simulink model "Pendel"  (Simulink 8.1)
settings: Solver=ode45  StartTime=0.0  StopTime=10.0  RelTol=1e-3
values from neighbouring files (symbols this model uses):
  dphi0 = 0    [Aufgabe_7_Loesung.m]
  dx0 = 0    [Aufgabe_7_Loesung.m]
  g = 9.81    [Aufgabe_7_Loesung.m]    (also in Aufgabe_8_Loesung.m)
  J_d = 5.8134e-4    (= 0.00058134)    [Aufgabe_7_Loesung.m]    (also in Aufgabe_8_Loesung.m)
  K = 1    [Aufgabe_7_Loesung.m]    (also in Aufgabe_8_Loesung.m)
  l_p = 0.147    [Aufgabe_7_Loesung.m]    (also in Aufgabe_8_Loesung.m)
  l_s = 0.5    [Aufgabe_7_Loesung.m]    (also in Aufgabe_8_Loesung.m)
  m_p = 0.0804    [Aufgabe_7_Loesung.m]    (also in Aufgabe_8_Loesung.m)
  mu = 8.5e-6    (= 8.5e-06)    [Aufgabe_7_Loesung.m]    (also in Aufgabe_8_Loesung.m)
  phi0 = 0    [Aufgabe_7_Loesung.m]
  T1 = 0.043    [Aufgabe_7_Loesung.m]    (also in Aufgabe_8_Loesung.m)
  Tt = 0.03    [Aufgabe_7_Loesung.m]    (also in Aufgabe_8_Loesung.m)
  x0 = 0    [Aufgabe_7_Loesung.m]
settings Model: Creator=St  LastModifiedBy=St
settings DataIOCC: SignalLoggingSaveFormat=Dataset
settings OptimizationCC: ExpressionDepthLimit=128
settings DebuggingCC: FcnCallInpInsideContextMsg=EnableAllAsError
settings GRTTargetCC: CombineOutputUpdateFcns=on  GRTInterface=off

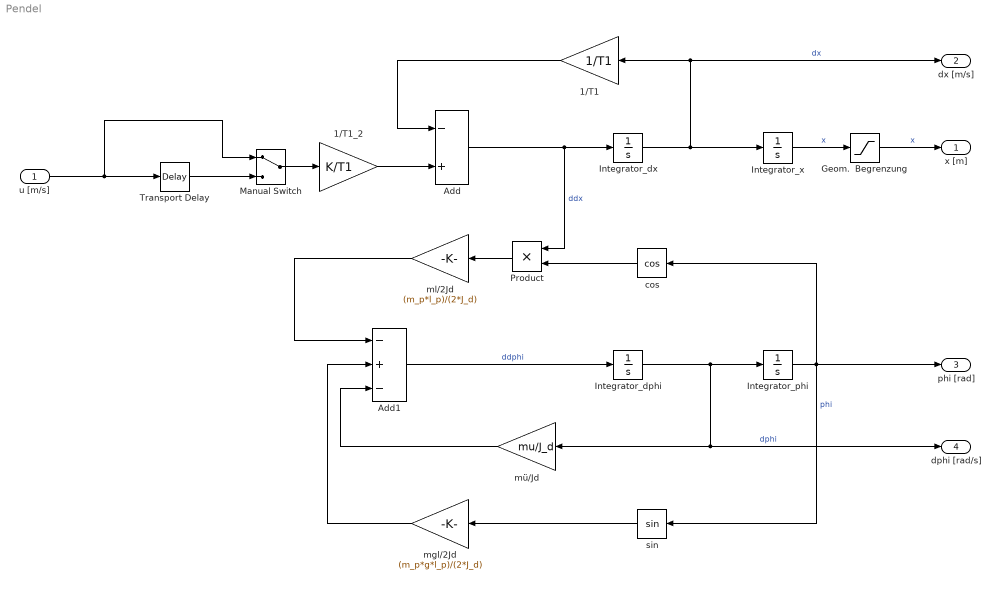
== system Pendel ==
  u [m/s] : Inport
  1/T1 : Gain  Gain=1/T1
  1/T1_2 : Gain  Gain=K/T1
  Add : Sum  Inputs=-+
  Add1 : Sum  Inputs=-+-
  Geom.  Begrenzung : Saturate  UpperLimit=l_s/2  LowerLimit=-l_s/2
  Integrator_dphi : Integrator  InitialCondition=dphi0
  Integrator_dx : Integrator  InitialCondition=dx0
  Integrator_phi : Integrator  InitialCondition=phi0
  Integrator_x : Integrator  InitialCondition=x0  UpperSaturationLimit=l_s/2  LowerSaturationLimit=-l_s/2
  Manual Switch : ManualSwitch
  Product : Product  RndMeth=Zero
  Transport Delay : TransportDelay  DelayTime=Tt
  cos : Trigonometry  Operator=cos
  mgl/2Jd : Gain  Gain=(m_p*g*l_p)/(2*J_d)
  ml/2Jd : Gain  Gain=(m_p*l_p)/(2*J_d)
  mü/Jd : Gain  Gain=mu/J_d
  sin : Trigonometry
  x [m] : Outport
  dx [m/s] : Outport  Port=2
  phi [rad] : Outport  Port=3
  dphi [rad/s] : Outport  Port=4
  wires:
  Integrator_dx/1 -> dx [m/s]/1, 1/T1/1, Integrator_x/1  "dx"
  Add/1 -> Integrator_dx/1, Product/1  "ddx"
  Integrator_x/1 -> Geom.  Begrenzung/1  "x"
  Integrator_dphi/1 -> mü/Jd/1, dphi [rad/s]/1, Integrator_phi/1  "dphi"
  Integrator_phi/1 -> cos/1, sin/1, phi [rad]/1  "phi"
  1/T1/1 -> Add/1
  mü/Jd/1 -> Add1/3
  cos/1 -> Product/2
  Product/1 -> ml/2Jd/1
  sin/1 -> mgl/2Jd/1
  mgl/2Jd/1 -> Add1/2
  Geom.  Begrenzung/1 -> x [m]/1  "x"
  Add1/1 -> Integrator_dphi/1  "ddphi"
  1/T1_2/1 -> Add/2
  ml/2Jd/1 -> Add1/1
  Manual Switch/1 -> 1/T1_2/1
  Transport Delay/1 -> Manual Switch/2
  u [m/s]/1 -> Manual Switch/1, Transport Delay/1
